simulink model "homework2"  (R2013a)
settings: Solver=ode45  StartTime=0.0  StopTime=10.0  RelTol=1e-6
StartFcn:
  | warning off
settings Model: Creator=OY  LastModifiedBy=mazzas

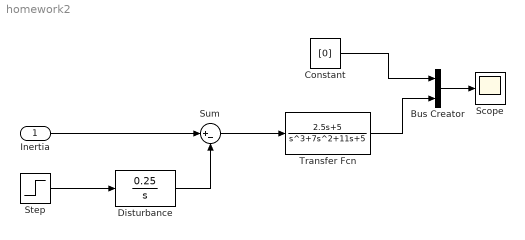
== system homework2 ==
  Inertia : Inport
  " Disturbance" : TransferFcn  Numerator=[0.25]  Denominator=[1 0]
  Bus Creator : BusCreator  Inputs=2
  Constant : Constant  Value=[0]
  Scope : Scope
  Step : Step  Time=0  SampleTime=0
  Sum : Sum  Inputs=|+-
  Transfer Fcn : TransferFcn  Numerator=[2.5 5]  Denominator=[1 7 11 5]
  wires:
  Transfer Fcn/1 -> Bus Creator/2
  Constant/1 -> Bus Creator/1
  Sum/1 -> Transfer Fcn/1
  Inertia/1 -> Sum/1
  Step/1 -> " Disturbance"/1
  " Disturbance"/1 -> Sum/2
  Bus Creator/1 -> Scope/1
